simulink model "kamasample1"  (R2014b)
settings: Solver=ode3  StartTime=0.0  StopTime=5  FixedStep=0.001  RelTol=1e-3
settings Model: Creator=zhoujie  LastModifiedBy=zhoujie

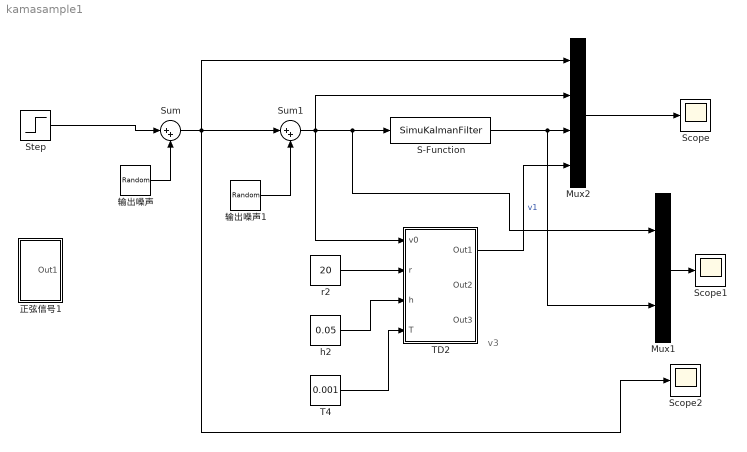
== system kamasample1 ==
  note: v3
  Mux1 : Mux  Inputs=2
  Mux2 : Mux
  S-Function : S-Function  FunctionName=SimuKalmanFilter  EnableBusSupport=off
  Scope : Scope
      settings: TimeRange=2.35610543302851  YMin=3.96022727272727  YMax=8.085227272727273
  Scope1 : Scope
      settings: TimeRange=2.35610543302851  YMin=3.96022727272727  YMax=8.085227272727273
  Scope2 : Scope
      settings: TimeRange=2.35610543302851  YMin=3.96022727272727  YMax=8.085227272727273  SaveName=ScopeData2
  Step : Step  After=0.3  SampleTime=0
  Sum : Sum  Inputs=|++
  Sum1 : Sum  Inputs=|++
  T4 : Constant  Value=0.001
  TD2 : Subsystem
  h2 : Constant  Value=0.05
  r2 : Constant  Value=20
  正弦信号1 : Subsystem
  输出噪声 : RandomNumber  Variance=0.001
  输出噪声1 : RandomNumber  Variance=0.001
  wires:
  输出噪声/1 -> Sum/2
  Sum/1 -> Scope2/1, Mux2/1, Sum1/1
  Mux2/1 -> Scope/1
  S-Function/1 -> Mux1/2, Mux2/3
  Sum1/1 -> Mux2/2, TD2/1(v0), Mux1/1, S-Function/1
  h2/1 -> TD2/3(h)
  r2/1 -> TD2/2(r)
  T4/1 -> TD2/4(T)
  TD2/1(Out1) -> Mux2/4  "v1"
  Mux1/1 -> Scope1/1
  Step/1 -> Sum/1
  输出噪声1/1 -> Sum1/2

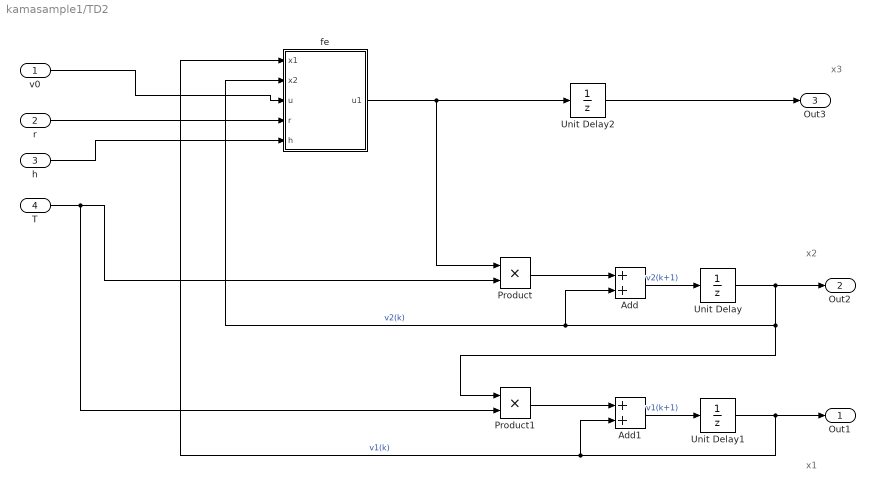
== system kamasample1/TD2 ==
  note: x3
  note: x2
  note: x1
  v0 : Inport
  r : Inport  Port=2
  h : Inport  Port=3
  T : Inport  Port=4
  Add : Sum
  Add1 : Sum
  Product : Product  RndMeth=Zero
  Product1 : Product  RndMeth=Zero
  Unit Delay : UnitDelay  SampleTime=-1
  Unit Delay1 : UnitDelay  SampleTime=-1
  Unit Delay2 : UnitDelay  SampleTime=-1
  fe : MATLAB Function  TreatAsAtomicUnit=on
  Out1 : Outport
  Out2 : Outport  Port=2
  Out3 : Outport  Port=3
  wires:
  v0/1 -> fe/3(u)
  r/1 -> fe/4(r)
  Product/1 -> Add/1
  Add/1 -> Unit Delay/1  "v2(k+1)"
  Unit Delay/1 -> fe/2(x2), Add/2, Product1/1, Out2/1  "v2(k)"
  Add1/1 -> Unit Delay1/1  "v1(k+1)"
  Unit Delay1/1 -> Out1/1, fe/1(x1), Add1/2  "v1(k)"
  Product1/1 -> Add1/1
  T/1 -> Product1/2, Product/2
  h/1 -> fe/5(h)
  fe/1(u1) -> Product/1, Unit Delay2/1
  Unit Delay2/1 -> Out3/1

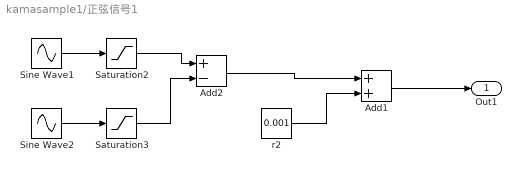
== system kamasample1/正弦信号1 ==
  Add1 : Sum
  Add2 : Sum  Inputs=+-
  Saturation2 : Saturate  UpperLimit=1  LowerLimit=0
  Saturation3 : Saturate  UpperLimit=0  LowerLimit=-1
  Sine Wave1 : Sin  Amplitude=0.3  Frequency=0.2  SampleTime=0
  Sine Wave2 : Sin  Amplitude=0.3  Frequency=0.2  SampleTime=0
  r2 : Constant  Value=0.001
  Out1 : Outport
  wires:
  Sine Wave2/1 -> Saturation3/1
  Sine Wave1/1 -> Saturation2/1
  Saturation2/1 -> Add2/1
  Saturation3/1 -> Add2/2
  Add1/1 -> Out1/1
  Add2/1 -> Add1/1
  r2/1 -> Add1/2

== matlab function kamasample1/TD2/fe ==
  data: x1 input; x2 input; u input; r input; h input; u1 output

function u1 = fhan(x1,x2,u,r,h)
delta = r*h; %h滤波因子  T跟踪步长  r为速度系数，r越大跟踪效果越好，但微分信号会增加高频噪声
delta0=delta*h;%反之，微分信号越平滑，会产生一定的滞后
b =x1-u+h*x2;
a0=sqrt(delta*delta+8*r*abs(b));
a=x2+b/h*(abs(b)<=delta0)+0.5*(a0-delta)*sign(b)*(abs(b)>delta0);
u1= -r*a/delta*(abs(a)<=delta)-r*sign(a)*(abs(a)>delta);
